simulink model "SBCAFinalSim"  (R2025b)
settings: Solver=FixedStepAuto  StartTime=0.0  StopTime=26  FixedStep=0.00005  MaxStep=0.1  RelTol=1e-3  AbsTol=1e-3  EnableMultiTasking=on
values from neighbouring files (symbols this model uses):
  K1 = lqr(A, B, Q, R_mat)    [Sim_Setup_Run_First.m]
  K2 = lqr(A, B, Q, R_mat)    [Sim_Setup_Run_First.m]
undefined symbols (not defined in the file or in its folder): X, Y, Z
libraries: sm_lib x18, nesl_utility x17
CloseFcn:
  | try,close(h1_sm_contact_ball),end
  | clear h1_sm_contact_ball
  | try,close(h2_sm_contact_ball),end
  | clear h2_sm_contact_ball
  | try,close(h3_sm_contact_ball),end
  | clear h3_sm_contact_ball
  | try,close(h4_sm_contact_ball),end
  | clear h4_sm_contact_ball
  | 
  | 
  | clear simlog_sm_contact_ball
  | clear logsout_sm_contact_ball
Description:
  | Bouncing Ball With Zero Crossings
  | 
  | Copyright 2019-2024 The MathWorks, Inc.
settings Model: Creator=smiller  LastModifiedBy=griffintrace
settings SolverCC: AutoScaleAbsTol=off  AlgebraicLoopSolver=TrustRegion  AutoInsertRateTranBlk=on
settings DataIOCC: LimitDataPoints=on  MaxDataPoints=10000  ReturnWorkspaceOutputs=off  SignalLoggingName=logsout_sm_contact_ball
settings OptimizationCC: ReuseModelBlockBuffer=off  LifeSpan=inf
settings DebuggingCC: UnconnectedInputMsg=warning  UnconnectedOutputMsg=warning  UnconnectedLineMsg=warning  AllowSymbolicDim=off  SFUnexpectedBacktrackingDiag=warning  SFNoUnconditionalDefaultTransitionDiag=warning  SFExecutionAtInitializationDiag=none  ArithmeticOperatorsInVariantConditions=warning
settings ModelReferenceCC: EnableRefExpFcnMdlSchedulingChecks=on
settings SFSimCC: SimUseLocalCustomCode=off  CustomCodeUndefinedFunction=UseInterfaceOnly
settings RTWCC: RTWUseLocalCustomCode=off  GPUComputeCapability=3.5  DLArmComputeVersion=19.05
settings CodeAppCC: StateflowObjectComments=on
settings GRTTargetCC: TargetLangStandard=C89/C90 (ANSI)
settings ConfigComp: CovMetricSettings=dw  CovSaveCumulativeToWorkspaceVar=on  CovSaveSingleToWorkspaceVar=on  CovExternalEMLEnable=off  CovSFcnEnable=off
settings SimscapeCC: SimscapeLogType=all  SimscapeLogSimulationStatistics=on  SimscapeLogName=simlog_sm_contact_ball  SimscapeLogDataHistory=10000.0
settings ExplorerConfigSet: InternalSimMechanicsExplorerSettings="<ExplorerConfiguration><canonicalview>default</canonicalview><AnimationSetting><BasePlaybackSpeed>1.0</BasePlaybackSpeed><PlaybackSpeedFactor>0.25</PlaybackSpeedFactor></AnimationSetting><TilePanel><TileInfo><Tiles Columns=\"1\" Count=\"2\" Rows=\"2\"><Column Weight=\"1\"/><Row Weight=\"0.5873\"/><Row Weight=\"0.4127\"/><Tile Height=\"1\" Width=\"1\" X=\"0\" Y=\"0\"/><Tile Height=\"1\" Width=\"1\" X=\"0\" Y=\"1\"/></Tiles></TileInfo><SceneInfo><SceneViewer><BGColor><R>1</R><G>1</G><B>1</B></BGColor><Camera><DoPerspective>off</DoPerspective><Position><X>-1.14521067233944529</X><Y>1.68242641303992024</Y><Z>0.238083627023966377</Z></Position><Center><X>-1.14521067233944529</X><Y>2.36058078639800328e-09</Y><Z>0.238083627023966377</Z></Center><Up><X>0</X><Y>0</Y><Z>1</Z></Up><ViewLimDist>1</ViewLimDist><YLim>0.433965796928594605</YLim><XLim>1.43706706523895278</XLim></Camera></SceneViewer><SceneViewer><BGColor><R>1</R><G>1</G><B>1</B></BGColor><Camera><DoPerspective>off</DoPerspective><Position><X>-1.14500851324288244</X><Y>0.00149877087782307591</Y><Z>1.68335583195827976</Z></Position><Center><X>-1.14500851324288244</X><Y>0.00149877087782307591</Y><Z>0.238083615161404305</Z></Center><Up><X>-0.00177367613036490167</X><Y>-0.9999984270352551</Y><Z>0</Z></Up><ViewLimDist>1</ViewLimDist><YLim>0.302405583873243622</YLim><XLim>1.43731595158576964</XLim></Camera></SceneViewer></SceneInfo></TilePanel><MechEditorPanel><Cameras/><GfxPanelCameraMap/><VideoCreator><PlaybackSpeedRatio>0.25</PlaybackSpeedRatio><FrameRate>30</FrameRate><VideoFormat>MPEG-4</VideoFormat><FrameSize>auto</FrameSize></VideoCreator></MechEditorPanel></ExplorerConfiguration>"

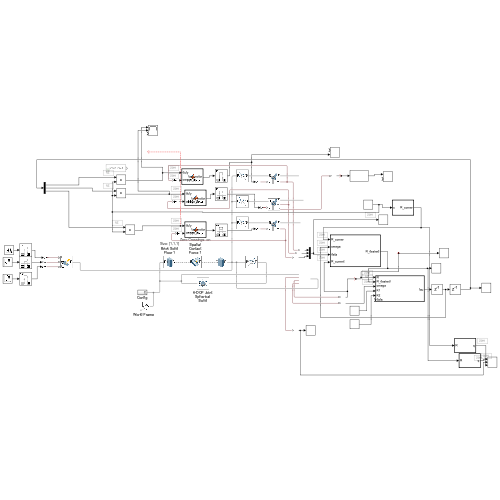
[thumbnail: Simulink's stored preview of the top-level diagram]
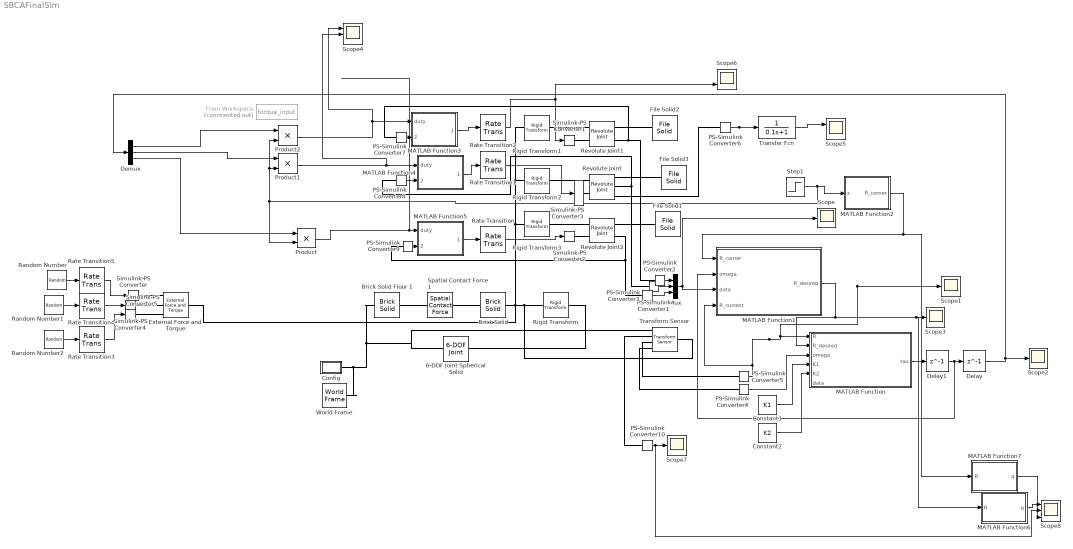
== system SBCAFinalSim ==
  6-DOF Joint Spherical Solid : sm_lib/Joints/6-DOF Joint  JointMode=Normal  CompositeWrenchDir=FollowerOnBase  CompositeWrenchFrame=BaseFrame  SenseConstraintForce=off  SenseConstraintTorque=off  SenseTotalForce=off  SenseTotalTorque=off  PxPositionTargetSpecify=off  PxPositionTargetPriority=High  PxPositionTargetValue=0  PxPositionTargetValueUnits=m  PxVelocityTargetSpecify=off  PxVelocityTargetPriority=High  PxVelocityTargetValue=0  PxVelocityTargetValueUnits=m/s  PxEquilibriumPosition=0  PxEquilibriumPositionUnits=m  PxSpringStiffness=0  PxSpringStiffnessUnits=N/m  PxDampingCoefficient=0  PxDampingCoefficientUnits=N/(m/s)  PxLowerLimitSpecify=off  PxLowerLimitBound=-1  PxLowerLimitBoundUnits=m  PxLowerLimitStiffness=1e6  PxLowerLimitStiffnessUnits=N/m  PxLowerLimitDamping=1e3  PxLowerLimitDampingUnits=N/(m/s)  PxLowerLimitTransitionRegionWidth=1e-4  PxLowerLimitTransitionRegionWidthUnits=m  PxUpperLimitSpecify=off  PxUpperLimitBound=1  PxUpperLimitBoundUnits=m  PxUpperLimitStiffness=1e6  PxUpperLimitStiffnessUnits=N/m  PxUpperLimitDamping=1e3  PxUpperLimitDampingUnits=N/(m/s)  PxUpperLimitTransitionRegionWidth=1e-4  PxUpperLimitTransitionRegionWidthUnits=m  PxTorqueActuationMode=NoTorque  PxMotionActuationMode=ComputedMotion  PxSensePosition=off  PxSenseVelocity=off  PxSenseAcceleration=off  PxSenseTorqueForce=off  PxSenseLowerLimitTorqueForce=off  PxSenseUpperLimitTorqueForce=off  PyPositionTargetSpecify=off  PyPositionTargetPriority=High  PyPositionTargetValue=0  PyPositionTargetValueUnits=m  PyVelocityTargetSpecify=off  PyVelocityTargetPriority=High  PyVelocityTargetValue=0  PyVelocityTargetValueUnits=m/s  PyEquilibriumPosition=0  PyEquilibriumPositionUnits=m  PySpringStiffness=0  PySpringStiffnessUnits=N/m  PyDampingCoefficient=0  PyDampingCoefficientUnits=N/(m/s)  PyLowerLimitSpecify=off  PyLowerLimitBound=-1  PyLowerLimitBoundUnits=m  PyLowerLimitStiffness=1e6  PyLowerLimitStiffnessUnits=N/m  PyLowerLimitDamping=1e3  PyLowerLimitDampingUnits=N/(m/s)  PyLowerLimitTransitionRegionWidth=1e-4  PyLowerLimitTransitionRegionWidthUnits=m  PyUpperLimitSpecify=off  PyUpperLimitBound=1  PyUpperLimitBoundUnits=m  PyUpperLimitStiffness=1e6  PyUpperLimitStiffnessUnits=N/m  PyUpperLimitDamping=1e3  PyUpperLimitDampingUnits=N/(m/s)  PyUpperLimitTransitionRegionWidth=1e-4  PyUpperLimitTransitionRegionWidthUnits=m  PyTorqueActuationMode=NoTorque  PyMotionActuationMode=ComputedMotion  PySensePosition=off  PySenseVelocity=off  PySenseAcceleration=off  PySenseTorqueForce=off  PySenseLowerLimitTorqueForce=off  PySenseUpperLimitTorqueForce=off  PzPositionTargetSpecify=on  PzPositionTargetPriority=High  PzPositionTargetValue=0.45  PzPositionTargetValueUnits=m  PzVelocityTargetSpecify=off  PzVelocityTargetPriority=High  PzVelocityTargetValue=0  PzVelocityTargetValueUnits=m/s  PzEquilibriumPosition=0  PzEquilibriumPositionUnits=m  PzSpringStiffness=0  PzSpringStiffnessUnits=N/m  PzDampingCoefficient=0  PzDampingCoefficientUnits=N/(m/s)  PzLowerLimitSpecify=off  PzLowerLimitBound=-1  PzLowerLimitBoundUnits=m  PzLowerLimitStiffness=1e6  PzLowerLimitStiffnessUnits=N/m  PzLowerLimitDamping=1e3  PzLowerLimitDampingUnits=N/(m/s)  PzLowerLimitTransitionRegionWidth=1e-4  PzLowerLimitTransitionRegionWidthUnits=m  PzUpperLimitSpecify=off  PzUpperLimitBound=1  PzUpperLimitBoundUnits=m  PzUpperLimitStiffness=1e6  PzUpperLimitStiffnessUnits=N/m  PzUpperLimitDamping=1e3  PzUpperLimitDampingUnits=N/(m/s)  PzUpperLimitTransitionRegionWidth=1e-4  PzUpperLimitTransitionRegionWidthUnits=m  PzTorqueActuationMode=NoTorque  PzMotionActuationMode=ComputedMotion  PzSensePosition=off  PzSenseVelocity=off  PzSenseAcceleration=off  PzSenseTorqueForce=off  PzSenseLowerLimitTorqueForce=off  PzSenseUpperLimitTorqueForce=off  SphPositionTargetSpecify=off  SphPositionTargetPriority=High  SphPositionTargetRotationMethod=None  SphPositionTargetFollAlignAxisA=+X  SphPositionTargetBaseAlignAxisA=+Y  SphPositionTargetFollAlignAxisB=+Y  SphPositionTargetBaseAlignAxisB=+Z  SphPositionTargetRotationStandardAxis=+Z  SphPositionTargetRotationAngle=0.0  SphPositionTargetRotationAngleUnits=deg  SphPositionTargetRotationArbitraryAxis=[0 0 1]  SphPositionTargetRotationSequenceAxes=FollowerAxes  SphPositionTargetRotationSequence=XYX  SphPositionTargetRotationSequenceAngles=[0 0 0]  SphPositionTargetRotationSequenceAnglesUnits=deg  SphPositionTargetRotationMatrix=[1 0 0; 0 1 0; 0 0 1]  SphPositionTargetQuaternion=[1 0 0 0]  SphVelocityTargetSpecify=off  SphVelocityTargetPriority=High  SphVelocityTargetValue=[0 0 0]  SphVelocityTargetValueUnits=deg/s  SphVelocityTargetInFollowerFrame=on  SphEqPosRotationMethod=None  SphEqPosFollAlignAxisA=+X  SphEqPosBaseAlignAxisA=+Y  SphEqPosFollAlignAxisB=+Y  SphEqPosBaseAlignAxisB=+Z  SphEqPosRotationStandardAxis=+Z  SphEqPosRotationAngle=0.0  SphEqPosRotationAngleUnits=deg  SphEqPosRotationArbitraryAxis=[0 0 1]  SphEqPosRotationSequenceAxes=FollowerAxes  SphEqPosRotationSequence=XYX  SphEqPosRotationSequenceAngles=[0 0 0]  SphEqPosRotationSequenceAnglesUnits=deg  SphEqPosRotationMatrix=[1 0 0; 0 1 0; 0 0 1]  SphEqPosQuaternion=[1 0 0 0]  SphSpringStiffness=0  SphSpringStiffnessUnits=N*m/deg  SphDampingCoefficient=0  SphDampingCoefficientUnits=N*m/(deg/s)  SphLowerLimitSpecify=off  SphLowerLimitBound=15  SphLowerLimitBoundUnits=deg  SphLowerLimitStiffness=1e4  SphLowerLimitStiffnessUnits=N*m/deg  SphLowerLimitDamping=10  SphLowerLimitDampingUnits=N*m/(deg/s)  SphLowerLimitTransitionRegionWidth=0.1  SphLowerLimitTransitionRegionWidthUnits=deg  SphUpperLimitSpecify=off  SphUpperLimitBound=45  SphUpperLimitBoundUnits=deg  SphUpperLimitStiffness=1e4  SphUpperLimitStiffnessUnits=N*m/deg  SphUpperLimitDamping=10  SphUpperLimitDampingUnits=N*m/(deg/s)  SphUpperLimitTransitionRegionWidth=0.1  SphUpperLimitTransitionRegionWidthUnits=deg  SphTorqueActuationMode=NoTorque  SphActuateTorqueX=off  SphActuateTorqueY=off  SphActuateTorqueZ=off  SphActuateTorque=off  SphActuationFrame=BaseFrame  SphSensePosition=off  SphSenseVelocityX=off  SphSenseVelocityY=off  SphSenseVelocityZ=off  SphSenseVelocity=off  SphSenseAccelerationX=off  SphSenseAccelerationY=off  SphSenseAccelerationZ=off  SphSenseAcceleration=off  SphSenseLowerLimitTorqueMag=off  SphSenseUpperLimitTorqueMag=off  SphSensingFrame=BaseFrame
  Brick Solid : sm_lib/Body Elements/Brick Solid  BrickDimensions=[0.124 0.124 0.124]  BrickDimensionsUnits=m  ExportEntireGeometry=on  InertiaType=Custom  BasedOnType=Mass  Density=1000  DensityUnits=kg/m^3  Mass=0.374  MassUnits=kg  CenterOfMass=[-20 -20 -20]  CenterOfMassUnits=mm  MomentsOfInertia=[0.0011441 0.0011441 0.0011441]  MomentsOfInertiaUnits=kg*m^2  ProductsOfInertia=[0.00018195 0.00018195 0.00018195]  ProductsOfInertiaUnits=kg*m^2  GraphicType=FromGeometry  MarkerShape=Sphere  MarkerSize=10  GraphicVisPropType=SimpleVisualProperties  GraphicDiffuseColor=[1 0 0]  GraphicOpacity=0.2  GraphicSpecularColor=[0.5 0.5 0.5 1.0]  GraphicAmbientColor=[0.15 0.15 0.15 1.0]  GraphicEmissiveColor=[0.0 0.0 0.0 1.0]  GraphicShininess=75  DoExposeReferenceFrame=on  SerializedFrames=<Frames/>
  Brick Solid Floor 1 : sm_lib/Body Elements/Brick Solid  BrickDimensions=[1,1,1]  BrickDimensionsUnits=m  ExportEntireGeometry=on  InertiaType=CalculateFromGeometry  BasedOnType=Density  Density=1000  DensityUnits=kg/m^3  Mass=1  MassUnits=kg  CenterOfMass=[0 0 0]  CenterOfMassUnits=m  MomentsOfInertia=[1 1 1]  MomentsOfInertiaUnits=kg*m^2  ProductsOfInertia=[0 0 0]  ProductsOfInertiaUnits=kg*m^2  GraphicType=FromGeometry  MarkerShape=Sphere  MarkerSize=10  GraphicVisPropType=SimpleVisualProperties  GraphicDiffuseColor=[0.7882 1 0.9725]  GraphicOpacity=1.0  GraphicSpecularColor=[0.5 0.5 0.5 1.0]  GraphicAmbientColor=[0.15 0.15 0.15 1.0]  GraphicEmissiveColor=[0.0 0.0 0.0 1.0]  GraphicShininess=75  DoExposeReferenceFrame=off  SerializedFrames=<Frames><Frame><Id>Frame1</Id><Value><Name>F1</Name><Origin><Source>ReferenceFrame</Source><FeatureName></FeatureName></Origin><PrimaryAxis><DefinedDirection>+Z</DefinedDirection><Source>ReferenceFrame</Source><SourceDirection>+Z</SourceDirection><FeatureName></FeatureName></PrimaryAxis><SecondaryAxis><DefinedDirection>+X</DefinedDirection><Source>ReferenceFrame</Source><SourceDirection>+X</SourceDirection><FeatureName></FeatureName></SecondaryAxis></Value></Frame></Frames>
      settings: AttributesFormatString=Size: %<BrickDimensions>
  Config : Subsystem
  Constant1 : Constant  Value=K1
  Constant2 : Constant  Value=K2
  Delay : Delay  DelayLength=1
  Delay1 : Delay  DelayLength=1
  Demux : Demux  Outputs=3
  External Force and Torque : sm_lib/Forces and Torques/External Force and Torque  EnableForceX=off  EnableForceY=off  EnableForceZ=off  EnableForce=off  ForceResolutionFrame=AttachedFrame  EnableTorqueX=on  EnableTorqueY=on  EnableTorqueZ=on  EnableTorque=off  TorqueResolutionFrame=AttachedFrame
  File Solid1 : sm_lib/Body Elements/File Solid  ExtGeomFileName=/Users/griffintrace/Downloads/Part Studio 1 - Wheel 1.step  UnitType=FromFile  ExtGeomFileUnits=m  StepReaderType=HEX  ExportConvexHullGeometry=off  InertiaType=Custom  BasedOnType=DensityFromFile  Density=1000  DensityUnits=kg/m^3  Mass=0.051  MassUnits=kg  CenterOfMass=[0 0 0]  CenterOfMassUnits=m  MomentsOfInertia=[0.00004749 0.00004749 0.00009362]  MomentsOfInertiaUnits=kg*m^2  ProductsOfInertia=[0 0 0]  ProductsOfInertiaUnits=kg*m^2  GraphicType=FromGeometry  MarkerShape=Sphere  MarkerSize=10  GraphicVisPropType=SimpleVisualProperties  GraphicDiffuseColor=[0.5 0.5 0.5]  GraphicOpacity=1  GraphicSpecularColor=[0.5 0.5 0.5 1.0]  GraphicAmbientColor=[0.15 0.15 0.15 1.0]  GraphicEmissiveColor=[0.0 0.0 0.0 1.0]  GraphicShininess=75  DoExposeReferenceFrame=on  SerializedFrames=<Frames/>
  File Solid2 : sm_lib/Body Elements/File Solid  ExtGeomFileName=/Users/griffintrace/Downloads/Part Studio 1 - Wheel 1.step  UnitType=FromFile  ExtGeomFileUnits=m  StepReaderType=HEX  ExportConvexHullGeometry=off  InertiaType=Custom  BasedOnType=DensityFromFile  Density=1000  DensityUnits=kg/m^3  Mass=0.051  MassUnits=kg  CenterOfMass=[0 0 0]  CenterOfMassUnits=m  MomentsOfInertia=[0.00004749 0.00004749 0.00009362]  MomentsOfInertiaUnits=kg*m^2  ProductsOfInertia=[0 0 0]  ProductsOfInertiaUnits=kg*m^2  GraphicType=FromGeometry  MarkerShape=Sphere  MarkerSize=10  GraphicVisPropType=SimpleVisualProperties  GraphicDiffuseColor=[0.5 0.5 0.5]  GraphicOpacity=1  GraphicSpecularColor=[0.5 0.5 0.5 1.0]  GraphicAmbientColor=[0.15 0.15 0.15 1.0]  GraphicEmissiveColor=[0.0 0.0 0.0 1.0]  GraphicShininess=75  DoExposeReferenceFrame=on  SerializedFrames=<Frames/>
  File Solid3 : sm_lib/Body Elements/File Solid  ExtGeomFileName=/Users/griffintrace/Downloads/Part Studio 1 - Wheel 1.step  UnitType=FromFile  ExtGeomFileUnits=m  StepReaderType=HEX  ExportConvexHullGeometry=off  InertiaType=Custom  BasedOnType=DensityFromFile  Density=1000  DensityUnits=kg/m^3  Mass=0.051  MassUnits=kg  CenterOfMass=[0 0 0]  CenterOfMassUnits=m  MomentsOfInertia=[0.00004749 0.00004749 0.00009362]  MomentsOfInertiaUnits=kg*m^2  ProductsOfInertia=[0 0 0]  ProductsOfInertiaUnits=kg*m^2  GraphicType=FromGeometry  MarkerShape=Sphere  MarkerSize=10  GraphicVisPropType=SimpleVisualProperties  GraphicDiffuseColor=[0.5 0.5 0.5]  GraphicOpacity=1  GraphicSpecularColor=[0.5 0.5 0.5 1.0]  GraphicAmbientColor=[0.15 0.15 0.15 1.0]  GraphicEmissiveColor=[0.0 0.0 0.0 1.0]  GraphicShininess=75  DoExposeReferenceFrame=on  SerializedFrames=<Frames/>
  From Workspace : FromWorkspace  Commented=on  VariableName=torque_input  SampleTime=-1
  MATLAB Function : MATLAB Function  TreatAsAtomicUnit=on  SystemSampleTime=0.0005
  MATLAB Function1 : MATLAB Function  TreatAsAtomicUnit=on  SystemSampleTime=0.001
  MATLAB Function2 : MATLAB Function  TreatAsAtomicUnit=on
  MATLAB Function3 : MATLAB Function  TreatAsAtomicUnit=on  SystemSampleTime=0.0001
  MATLAB Function4 : MATLAB Function  TreatAsAtomicUnit=on  SystemSampleTime=0.0001
  MATLAB Function5 : MATLAB Function  TreatAsAtomicUnit=on  SystemSampleTime=0.0001
  MATLAB Function6 : MATLAB Function  TreatAsAtomicUnit=on
  MATLAB Function7 : MATLAB Function  TreatAsAtomicUnit=on
  Mux : Mux  Inputs=3
  PS-Simulink Converter{1..10} (10 alike) : nesl_utility/PS-Simulink Converter  PhysicalDomain=network_engine_domain  SubClassName=ps_output  LeftPortType=input  RightPortType=output  PseudoPeriodic=off  Frequencies=[]  VectorFormat=inherit  Unit=inherit  AffineConversion=off
  Product : Product
  Product1 : Product
  Product2 : Product
  Random Number : RandomNumber  Variance=0.01  SampleTime=0.001
  Random Number1 : RandomNumber  Variance=0.01  Seed=10000  SampleTime=0.001
  Random Number2 : RandomNumber  Variance=0.01  Seed=10  SampleTime=0.001
  Rate Transition{,1..5} (6 alike) : RateTransition
  Revolute Joint : sm_lib/Joints/Revolute Joint  JointMode=Normal  CompositeWrenchDir=FollowerOnBase  CompositeWrenchFrame=BaseFrame  SenseConstraintForce=off  SenseConstraintTorque=off  SenseTotalForce=off  SenseTotalTorque=off  PositionTargetSpecify=off  PositionTargetPriority=High  PositionTargetValue=0  PositionTargetValueUnits=deg  VelocityTargetSpecify=off  VelocityTargetPriority=High  VelocityTargetValue=0  VelocityTargetValueUnits=deg/s  EquilibriumPosition=0  EquilibriumPositionUnits=deg  SpringStiffness=0  SpringStiffnessUnits=N*m/deg  DampingCoefficient=0  DampingCoefficientUnits=N*m/(deg/s)  LowerLimitSpecify=off  LowerLimitBound=-90  LowerLimitBoundUnits=deg  LowerLimitStiffness=1e4  LowerLimitStiffnessUnits=N*m/deg  LowerLimitDamping=10  LowerLimitDampingUnits=N*m/(deg/s)  LowerLimitTransitionRegionWidth=0.1  LowerLimitTransitionRegionWidthUnits=deg  UpperLimitSpecify=off  UpperLimitBound=90  UpperLimitBoundUnits=deg  UpperLimitStiffness=1e4  UpperLimitStiffnessUnits=N*m/deg  UpperLimitDamping=10  UpperLimitDampingUnits=N*m/(deg/s)  UpperLimitTransitionRegionWidth=0.1  UpperLimitTransitionRegionWidthUnits=deg  TorqueActuationMode=InputTorque  MotionActuationMode=ComputedMotion  SensePosition=off  SenseVelocity=on  SenseAcceleration=off  SenseTorqueForce=on  SenseLowerLimitTorqueForce=off  SenseUpperLimitTorqueForce=off
  Revolute Joint1 : sm_lib/Joints/Revolute Joint  JointMode=Normal  CompositeWrenchDir=FollowerOnBase  CompositeWrenchFrame=BaseFrame  SenseConstraintForce=off  SenseConstraintTorque=off  SenseTotalForce=off  SenseTotalTorque=off  PositionTargetSpecify=off  PositionTargetPriority=High  PositionTargetValue=0  PositionTargetValueUnits=deg  VelocityTargetSpecify=off  VelocityTargetPriority=High  VelocityTargetValue=0  VelocityTargetValueUnits=deg/s  EquilibriumPosition=0  EquilibriumPositionUnits=deg  SpringStiffness=0  SpringStiffnessUnits=N*m/deg  DampingCoefficient=0  DampingCoefficientUnits=N*m/(deg/s)  LowerLimitSpecify=off  LowerLimitBound=-90  LowerLimitBoundUnits=deg  LowerLimitStiffness=1e4  LowerLimitStiffnessUnits=N*m/deg  LowerLimitDamping=10  LowerLimitDampingUnits=N*m/(deg/s)  LowerLimitTransitionRegionWidth=0.1  LowerLimitTransitionRegionWidthUnits=deg  UpperLimitSpecify=off  UpperLimitBound=90  UpperLimitBoundUnits=deg  UpperLimitStiffness=1e4  UpperLimitStiffnessUnits=N*m/deg  UpperLimitDamping=10  UpperLimitDampingUnits=N*m/(deg/s)  UpperLimitTransitionRegionWidth=0.1  UpperLimitTransitionRegionWidthUnits=deg  TorqueActuationMode=InputTorque  MotionActuationMode=ComputedMotion  SensePosition=off  SenseVelocity=on  SenseAcceleration=off  SenseTorqueForce=off  SenseLowerLimitTorqueForce=off  SenseUpperLimitTorqueForce=off
  Revolute Joint2 : sm_lib/Joints/Revolute Joint  JointMode=Normal  CompositeWrenchDir=FollowerOnBase  CompositeWrenchFrame=BaseFrame  SenseConstraintForce=off  SenseConstraintTorque=off  SenseTotalForce=off  SenseTotalTorque=off  PositionTargetSpecify=off  PositionTargetPriority=High  PositionTargetValue=0  PositionTargetValueUnits=deg  VelocityTargetSpecify=off  VelocityTargetPriority=High  VelocityTargetValue=0  VelocityTargetValueUnits=deg/s  EquilibriumPosition=0  EquilibriumPositionUnits=deg  SpringStiffness=0  SpringStiffnessUnits=N*m/deg  DampingCoefficient=0  DampingCoefficientUnits=N*m/(deg/s)  LowerLimitSpecify=off  LowerLimitBound=-90  LowerLimitBoundUnits=deg  LowerLimitStiffness=1e4  LowerLimitStiffnessUnits=N*m/deg  LowerLimitDamping=10  LowerLimitDampingUnits=N*m/(deg/s)  LowerLimitTransitionRegionWidth=0.1  LowerLimitTransitionRegionWidthUnits=deg  UpperLimitSpecify=off  UpperLimitBound=90  UpperLimitBoundUnits=deg  UpperLimitStiffness=1e4  UpperLimitStiffnessUnits=N*m/deg  UpperLimitDamping=10  UpperLimitDampingUnits=N*m/(deg/s)  UpperLimitTransitionRegionWidth=0.1  UpperLimitTransitionRegionWidthUnits=deg  TorqueActuationMode=InputTorque  MotionActuationMode=ComputedMotion  SensePosition=off  SenseVelocity=on  SenseAcceleration=off  SenseTorqueForce=off  SenseLowerLimitTorqueForce=off  SenseUpperLimitTorqueForce=off
  Rigid Transform : sm_lib/Frames and Transforms/Rigid Transform  RotationMethod=StandardAxis  FollAlignAxisA=+X  BaseAlignAxisA=+Y  FollAlignAxisB=+Y  BaseAlignAxisB=+Z  RotationStandardAxis=+Y  RotationAngle=0  RotationAngleUnits=deg  RotationArbitraryAxis=[0 0 1]  RotationSequenceAxes=FollowerAxes  RotationSequence=XYX  RotationSequenceAngles=[0 0 0]  RotationSequenceAnglesUnits=deg  RotationMatrix=[1 0 0;0 1 0;0 0 1]  Quaternion=[1 0 0 0]  TranslationMethod=StandardAxis  TranslationCartesianOffset=[0 0 0]  TranslationCartesianOffsetUnits=m  TranslationStandardAxis=+Z  TranslationStandardOffset=-0.112  TranslationStandardOffsetUnits=m  TranslationROffset=0  TranslationROffsetUnits=m  TranslationThetaOffset=0  TranslationThetaOffsetUnits=deg  TranslationZOffset=0  TranslationZOffsetUnits=m
  Rigid Transform1 : sm_lib/Frames and Transforms/Rigid Transform  RotationMethod=StandardAxis  FollAlignAxisA=+X  BaseAlignAxisA=+Y  FollAlignAxisB=+Y  BaseAlignAxisB=+Z  RotationStandardAxis=-Y  RotationAngle=90  RotationAngleUnits=deg  RotationArbitraryAxis=[0 0 1]  RotationSequenceAxes=FollowerAxes  RotationSequence=XYX  RotationSequenceAngles=[0 0 0]  RotationSequenceAnglesUnits=deg  RotationMatrix=[1 0 0;0 1 0;0 0 1]  Quaternion=[1 0 0 0]  TranslationMethod=Cartesian  TranslationCartesianOffset=[0 0 0.055]  TranslationCartesianOffsetUnits=m  TranslationStandardAxis=+Z  TranslationStandardOffset=0  TranslationStandardOffsetUnits=m  TranslationROffset=0  TranslationROffsetUnits=m  TranslationThetaOffset=0  TranslationThetaOffsetUnits=deg  TranslationZOffset=0  TranslationZOffsetUnits=m
  Rigid Transform2 : sm_lib/Frames and Transforms/Rigid Transform  RotationMethod=StandardAxis  FollAlignAxisA=+X  BaseAlignAxisA=+Y  FollAlignAxisB=+Y  BaseAlignAxisB=+Z  RotationStandardAxis=+X  RotationAngle=90  RotationAngleUnits=deg  RotationArbitraryAxis=[0 0 1]  RotationSequenceAxes=FollowerAxes  RotationSequence=XYX  RotationSequenceAngles=[0 0 0]  RotationSequenceAnglesUnits=deg  RotationMatrix=[1 0 0;0 1 0;0 0 1]  Quaternion=[1 0 0 0]  TranslationMethod=Cartesian  TranslationCartesianOffset=[0 0 0.055]  TranslationCartesianOffsetUnits=m  TranslationStandardAxis=+Z  TranslationStandardOffset=0  TranslationStandardOffsetUnits=m  TranslationROffset=0  TranslationROffsetUnits=m  TranslationThetaOffset=0  TranslationThetaOffsetUnits=deg  TranslationZOffset=0  TranslationZOffsetUnits=m
  Rigid Transform3 : sm_lib/Frames and Transforms/Rigid Transform  RotationMethod=StandardAxis  FollAlignAxisA=+X  BaseAlignAxisA=+Y  FollAlignAxisB=+Y  BaseAlignAxisB=+Z  RotationStandardAxis=-Z  RotationAngle=90  RotationAngleUnits=deg  RotationArbitraryAxis=[0 0 1]  RotationSequenceAxes=FollowerAxes  RotationSequence=XYX  RotationSequenceAngles=[0 0 0]  RotationSequenceAnglesUnits=deg  RotationMatrix=[1 0 0;0 1 0;0 0 1]  Quaternion=[1 0 0 0]  TranslationMethod=Cartesian  TranslationCartesianOffset=[0 0 0.055]  TranslationCartesianOffsetUnits=m  TranslationStandardAxis=+Z  TranslationStandardOffset=0  TranslationStandardOffsetUnits=m  TranslationROffset=0  TranslationROffsetUnits=m  TranslationThetaOffset=0  TranslationThetaOffsetUnits=deg  TranslationZOffset=0  TranslationZOffsetUnits=m
  Scope{,1..3,7} (5 alike) : Scope
      Scope settings: SampleTime=0.01  ActiveDisplayYMinimum=-606.88398  ActiveDisplayYMaximum=752.93887  DataLoggingVariableName=RPM
      Scope1 settings: ActiveDisplayYMinimum=-0.95959  ActiveDisplayYMaximum=1.21773  DataLoggingVariableName=ScopeData2
      Scope2 settings: ActiveDisplayYMinimum=-1.25  ActiveDisplayYMaximum=1.25
      Scope3 settings: ActiveDisplayYMinimum=-1.78359  ActiveDisplayYMaximum=1.88444  DataLoggingVariableName=ScopeData3
      Scope7 settings: ActiveDisplayYMinimum=-1.25  ActiveDisplayYMaximum=1.25
  Scope4 : Scope  NumInputPorts=3
      settings: ActiveDisplayYMinimum=-0.125  ActiveDisplayYMaximum=1.125
  Scope5 : Scope  NumInputPorts=2
      settings: ActiveDisplayYMinimum=-0.79406  ActiveDisplayYMaximum=0.62384  DataLoggingVariableName=ScopeData2
  Scope6 : Scope  NumInputPorts=2
      settings: ActiveDisplayYMinimum=-0.3668  ActiveDisplayYMaximum=0.36762  DataLoggingVariableName=ScopeData3
  Scope8 : Scope  NumInputPorts=3
      settings: SampleTime=0.01  ActiveDisplayYMinimum=-0.61104  ActiveDisplayYMaximum=1.179  DataLoggingVariableName=PosSim
  Simulink-PS Converter : nesl_utility/Simulink-PS Converter  PhysicalDomain=network_engine_domain  SubClassName=ps_input  LeftPortType=input  RightPortType=output  PseudoPeriodic=off  Frequencies=[]  NoiseDistribution=none  NoiseParameters=[]  Unit=1  AffineConversion=off  FilteringAndDerivatives=filter  SimscapeFilterOrder=1  InputFilterTimeConstant=0.1  UdotUserProvided=0
  Simulink-PS Converter1 : nesl_utility/Simulink-PS Converter  PhysicalDomain=network_engine_domain  SubClassName=ps_input  LeftPortType=input  RightPortType=output  PseudoPeriodic=off  Frequencies=[]  NoiseDistribution=none  NoiseParameters=[]  Unit=1  AffineConversion=off  FilteringAndDerivatives=provide  SimscapeFilterOrder=2  InputFilterTimeConstant=0.0001  UdotUserProvided=0
  Simulink-PS Converter2 : nesl_utility/Simulink-PS Converter  PhysicalDomain=network_engine_domain  SubClassName=ps_input  LeftPortType=input  RightPortType=output  PseudoPeriodic=off  Frequencies=[]  NoiseDistribution=none  NoiseParameters=[]  Unit=1  AffineConversion=off  FilteringAndDerivatives=provide  SimscapeFilterOrder=2  InputFilterTimeConstant=0.0001  UdotUserProvided=0
  Simulink-PS Converter3 : nesl_utility/Simulink-PS Converter  PhysicalDomain=network_engine_domain  SubClassName=ps_input  LeftPortType=input  RightPortType=output  PseudoPeriodic=off  Frequencies=[]  NoiseDistribution=none  NoiseParameters=[]  Unit=1  AffineConversion=off  FilteringAndDerivatives=provide  SimscapeFilterOrder=2  InputFilterTimeConstant=0.0001  UdotUserProvided=0
  Simulink-PS Converter4 : nesl_utility/Simulink-PS Converter  PhysicalDomain=network_engine_domain  SubClassName=ps_input  LeftPortType=input  RightPortType=output  PseudoPeriodic=off  Frequencies=[]  NoiseDistribution=none  NoiseParameters=[]  Unit=1  AffineConversion=off  FilteringAndDerivatives=filter  SimscapeFilterOrder=1  InputFilterTimeConstant=0.1  UdotUserProvided=0
  Simulink-PS Converter5 : nesl_utility/Simulink-PS Converter  PhysicalDomain=network_engine_domain  SubClassName=ps_input  LeftPortType=input  RightPortType=output  PseudoPeriodic=off  Frequencies=[]  NoiseDistribution=none  NoiseParameters=[]  Unit=1  AffineConversion=off  FilteringAndDerivatives=filter  SimscapeFilterOrder=1  InputFilterTimeConstant=0.1  UdotUserProvided=0
  Spatial Contact Force 1 : sm_lib/Forces and Torques/Spatial Contact Force  SenseSeparationDistance=off  NormalForceType=SmoothSpringDamper  NormalStiffness=1e7  NormalStiffnessUnits=N/m  NormalDamping=10e3  NormalDampingUnits=N/(m/s)  NormalTransitionRegionWidth=5e-2  NormalTransitionRegionWidthUnits=m  FrictionType=SmoothStickSlip  CoefficientOfStaticFriction=1  CoefficientOfDynamicFriction=1  FrictionalCriticalVelocity=1e-3  FrictionalCriticalVelocityUnits=m/s  SenseContactSignal=off  SensePenetrationDepth=off  SenseNormalVelocity=off  SenseTangentialVelocity=off  SensingForceTorqueDirection=BaseOnFollower  SensingForceTorqueResolutionFrame=ContactFrame  SenseNormalForce=off  SenseNormalForceMagnitude=off  SenseNormalTorque=off  SenseFrictionalForce=off  SenseFrictionalForceMagnitude=off  SenseFrictionalTorque=off  SenseTotalForce=off  SenseTotalTorque=off  SenseContactBaseRotation=off  SenseContactBaseTranslation=off  SenseContactFollowerRotation=off  SenseContactFollowerTranslation=off  ZeroCrossDetectContactStartAndEnd=on
      settings: AttributesFormatString=Zero Crossings: %<ZeroCrossDetectContactStartAndEnd>
  Step1 : Step  SampleTime=0
  Transfer Fcn : TransferFcn  Denominator=[0.1 1]
  Transform Sensor : sm_lib/Frames and Transforms/Transform Sensor  MeasurementFrame=World  RotationSequence=XYZ  SenseAngle=off  SenseAxis=off  SenseQ=on  SenseR=on  SenseRotationSequence=off  SenseOmegaX=off  SenseOmegaY=off  SenseOmegaZ=off  SenseOmega=on  SenseQDot=off  SenseRDot=off  SenseRotationSequenceDot=off  SenseAlphaX=off  SenseAlphaY=off  SenseAlphaZ=off  SenseAlpha=off  SenseQDDot=off  SenseRDDot=off  SenseX=off  SenseY=off  SenseZ=off  SenseXYZ=off  SenseRad=off  SenseAzim=off  SenseDist=off  SenseInc=off  SenseXDot=off  SenseYDot=off  SenseZDot=off  SenseXYZDot=off  SenseRadDot=off  SenseAzimDot=off  SenseDistDot=off  SenseIncDot=off  SenseXDDot=off  SenseYDDot=off  SenseZDDot=off  SenseXYZDDot=off  SenseRadDDot=off  SenseAzimDDot=off  SenseDistDDot=off  SenseIncDDot=off
  World Frame : sm_lib/Frames and Transforms/World Frame
  wires:
  PS-Simulink Converter1/1 -> Mux/2
  PS-Simulink Converter5/1 -> Scope1/1, MATLAB Function/1(R), MATLAB Function1/4(R_current)
  Mux/1 -> Scope/1, MATLAB Function1/3(data)
  PS-Simulink Converter2/1 -> Mux/1
  PS-Simulink Converter3/1 -> Mux/3
  PS-Simulink Converter4/1 -> MATLAB Function/3(omega)
  MATLAB Function1/1(R_desired) -> MATLAB Function/2(R_desired), MATLAB Function6/1(R), Scope3/1
  MATLAB Function2/1(R_corner) -> MATLAB Function7/1(R), MATLAB Function1/1(R_corner)
  Step1/1 -> Product/2, Product1/2, Product2/2, MATLAB Function2/1(x)
  MATLAB Function3/1(tau_motor) -> Rate Transition2/1
  Rate Transition/1 -> Simulink-PS Converter2/1
  Rate Transition2/1 -> Simulink-PS Converter1/1, Scope6/2
  MATLAB Function4/1(tau_motor) -> Rate Transition1/1
  MATLAB Function5/1(tau_motor) -> Rate Transition/1
  PS-Simulink Converter6/1 -> Transfer Fcn/1
  Rate Transition1/1 -> Simulink-PS Converter3/1
  Transfer Fcn/1 -> Scope5/1
  PS-Simulink Converter7/1 -> MATLAB Function3/2(omega_w)
  PS-Simulink Converter8/1 -> MATLAB Function4/2(omega_w)
  PS-Simulink Converter9/1 -> MATLAB Function5/2(omega_w)
  PS-Simulink Converter10/1 -> Scope8/2, Scope7/1
  Delay/1 -> Demux/1, Scope2/1
  Demux/3 -> Product/1
  Demux/2 -> Product1/1
  Demux/1 -> Product2/1
  Product2/1 -> Scope4/1, MATLAB Function3/1(duty)
  Product1/1 -> MATLAB Function4/1(duty), Scope4/2
  Product/1 -> MATLAB Function5/1(duty)
  Constant1/1 -> MATLAB Function/4(K1)
  Constant2/1 -> MATLAB Function/5(K2)
  Delay1/1 -> MATLAB Function1/2(omega), Delay/1
  MATLAB Function/1(tau) -> Delay1/1
  Random Number/1 -> Rate Transition5/1
  Random Number1/1 -> Rate Transition4/1
  Random Number2/1 -> Rate Transition3/1
  Rate Transition3/1 -> Simulink-PS Converter5/1
  Rate Transition4/1 -> Simulink-PS Converter4/1
  Rate Transition5/1 -> Simulink-PS Converter/1
  MATLAB Function6/1(q) -> Scope8/1
  MATLAB Function7/1(q) -> Scope8/3
  connections:
  World Frame/RConn1 -- 6-DOF Joint Spherical Solid/LConn1 -- Transform Sensor/RConn1 -- Brick Solid Floor 1/LConn1 -- Config/RConn1
  Spatial Contact Force 1/RConn1 -- Brick Solid/LConn1
  Rigid Transform/LConn1 -- External Force and Torque/RConn1 -- Brick Solid/RConn1 -- Rigid Transform3/RConn1 -- Rigid Transform1/RConn1 -- Rigid Transform2/RConn1 -- Transform Sensor/LConn1
  Rigid Transform/RConn1 -- 6-DOF Joint Spherical Solid/RConn1
  Brick Solid Floor 1/RConn1 -- Spatial Contact Force 1/LConn1
  File Solid3/RConn1 -- Revolute Joint/RConn1
  Simulink-PS Converter3/RConn1 -- Revolute Joint/LConn2
  Revolute Joint/RConn2 -- PS-Simulink Converter8/LConn1 -- PS-Simulink Converter1/LConn1
  Rigid Transform2/LConn1 -- Revolute Joint/LConn1
  Transform Sensor/RConn3 -- PS-Simulink Converter5/LConn1
  Transform Sensor/RConn4 -- PS-Simulink Converter4/LConn1
  File Solid2/RConn1 -- Revolute Joint1/RConn1
  Rigid Transform1/LConn1 -- Revolute Joint1/LConn1
  PS-Simulink Converter2/LConn1 -- PS-Simulink Converter7/LConn1 -- Revolute Joint1/RConn2
  Simulink-PS Converter1/RConn1 -- Revolute Joint1/LConn2
  File Solid1/RConn1 -- Revolute Joint2/RConn1
  Rigid Transform3/LConn1 -- Revolute Joint2/LConn1
  Revolute Joint2/RConn2 -- PS-Simulink Converter9/LConn1 -- PS-Simulink Converter3/LConn1
  Simulink-PS Converter2/RConn1 -- Revolute Joint2/LConn2
  Revolute Joint/RConn3 -- PS-Simulink Converter6/LConn1
  Transform Sensor/RConn2 -- PS-Simulink Converter10/LConn1
  Simulink-PS Converter/RConn1 -- External Force and Torque/LConn1
  Simulink-PS Converter5/RConn1 -- External Force and Torque/LConn3
  Simulink-PS Converter4/RConn1 -- External Force and Torque/LConn2

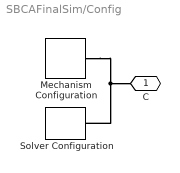
== system SBCAFinalSim/Config ==
  Mechanism Configuration : sm_lib/Utilities/Mechanism Configuration  UniformGravity=Constant  GravityVector=[0 0 -9.80665]  GravityVectorUnits=m/s^2  LinearizationDelta=0.001  JointModeTransitionNonlinearIterations=2
  Solver Configuration : nesl_utility/Solver Configuration  PhysicalDomain=network_engine_domain  SubClassName=solver  LeftPortType=input  RightPortType=generic  Tones=[]  Harmonics=[]  SimulateNoise=off  Profile=off  UseLocalSampling=off  EnableSwitchedLinearOptims=on  FrequencyDomain=off  UseCCode=off  RelTol=0.001  AbsTol=1e-06  MinStep=1e-09  ToWorkspace=off  RevertToSquareIcSolve=off  NumHomotopyIterations=100  PhasorMode=off  PhasorModeNumHarmonics=1  ConsistencySolver=NEWTON_FTOL  IndexReductionMethod=DerivativeReplacement  DoDC=off  ResidualTolerance=1e-09  ConsistencyTolSource=GLOBAL  ConsistencyAbsTol=0.001  ConsistencyRelTol=0.001  ConsistencyTolFactor=0.001  UseLocalSolver=off  LocalSolverChoice=NE_BACKWARD_EULER_ADVANCER  ResolveIndetEquations=on  FunctionEvalNumThread=1  LocalSolverSampleTime=0.001  DoFixedCost=off  MaxNonlinIter=3  MaxModeIter=2  ComputeImpulses=off  ImpulseIterations=2  LinearAlgebra=Sparse  LinearAlgebraNumThread=0  EquationFormulation=NE_TIME_EF  DelaysMemoryBudget=1024  AutomaticFiltering=on  FilteringTimeConstant=0.001  PartitionStorageMethod=AS_NEEDED  PartitionMemoryBudget=1024  PartitionMethod=FAST  MultibodyUseLocalSolver=off  MultibodyLocalSolverChoice=ODE1  MultibodyLocalSolverSampleTime=0.001
  C : PMIOPort  Side=Right
  connections:
  Mechanism Configuration/RConn1 -- Solver Configuration/RConn1 -- C/RConn1

== matlab function SBCAFinalSim/MATLAB Function1 ==
  settings: updateMethod=DISCRETE
  data: R_corner input; R_desired output; omega input; data input; R_current input
function R_desired = despool_tilt_controller(R_corner, omega, data, R_current)
% despool_tilt_controller - Tilt R_corner up to 10 deg in direction of omega*R_current
%
% Inputs:
%   R_corner  - 3x3 rotation matrix of cube balanced on corner (fixed setpoint)
%   omega     - 3x1 angular velocity vector in body frame
%   R_current - 3x3 current rotation matrix (body-to-world)
%
% Output:
%   R_desired - 3x3 desired rotation matrix (tilted setpoint)

    % Apply bias to omega
    omega = omega -[-0.1;0.1;-0.1];
    persistent omega_smooth initialized
alpha = 0.005;  % smoothing factor (tune between 0.005)

if isempty(initialized)
    omega_smooth = omega;   % initialize
    initialized = true;
end

omega_smooth = (1 - alpha) * omega_smooth + alpha * omega;

omega = omega_smooth; 
%omega=omega-mean(omega);
omega = sign(omega).*abs(omega).^2+omega;
omega = max(min(omega, 0.4), -0.4);
    

    tilt_axis_world =  eulerToR(omega/2);

    R_desired = tilt_axis_world  * R_corner;
end

function R = axisAngleToRotationMatrix(axis, angle)
    % Rodrigues' rotation formula
    axis = axis / norm(axis);
    K = [  0       -axis(3)  axis(2);
          axis(3)     0     -axis(1);
         -axis(2)  axis(1)     0  ];
    R = eye(3) + sin(angle) * K + (1 - cos(angle)) * (K * K);
end
function R = eulerToR(omega)
% omega = [roll; pitch; yaw] in radians

    roll  = omega(1);
    pitch = omega(2);
    yaw   = omega(3);

    Rx = [1, 0, 0;
          0, cos(roll), -sin(roll);
          0, sin(roll),  cos(roll)];

    Ry = [ cos(pitch), 0, sin(pitch);
           0, 1, 0;
          -sin(pitch), 0, cos(pitch)];

    Rz = [cos(yaw), -sin(yaw), 0;
          sin(yaw),  cos(yaw), 0;
          0, 0, 1];

    % Final combined rotation
    R = Rz * Ry * Rx;
end

== matlab function SBCAFinalSim/MATLAB Function ==
  settings: updateMethod=DISCRETE
  data: R input; R_desired input; omega input; tau output; K1 input; K2 input; data input
function tau = balanceCubeLQR(R, R_desired, omega, K1, K2, data)
% balanceCubeLQR - Computes torque using angle-dependent LQR with smooth transition
%
% Inputs:
%   R         - Current rotation matrix (3x3)
%   R_desired - Desired rotation matrix (3x3)
%   omega     - Angular velocity in body frame (3x1)
%   K1        - LQR gain matrix for small error (3x6)
%   K2        - LQR gain matrix for large error (3x6)
%
% Output:
%   tau       - Torque command (3x1)

    % Compute state vector
    x = computeStateVector(R, R_desired, omega);

    % --- Compute misalignment angle between R and R_desired ---
    R_err = R_desired' * R;
    cos_theta = (trace(R_err) - 1) / 2;
    cos_theta = max(min(cos_theta, 1), -1);  % numerical safety
    angle_err_mag = acosd(cos_theta);        % in degrees

    % --- Blended gain selection ---
    if angle_err_mag <= 10
        alpha = 0;   % fully K1
    elseif angle_err_mag >= 25
        alpha = 1;   % fully K2
    else
        % Linear blend between 5° and 10°
        alpha = (angle_err_mag - 10) / 15;
    end


    

    % --- LQR torque command ---
    tau = -K1 * x.*alpha-K2*x.*(1-alpha);%+[0.05;-0.05;0.05];

    % --- Torque saturation ---
    max_tau = 1;  % Adjust based on motor/wheel limits
    tau = max(min(tau, max_tau), -max_tau);
    alpha1 = 0.5;
    persistent tau_prev
if isempty(tau_prev)
    tau_prev = zeros(size(tau));
end

tau_out = tau;
for i = 1:numel(tau)
    if abs(tau) < abs(tau_prev)
        tau_out = alpha1 * tau + (1 - alpha1) * tau_prev;
    end
end
tau=tau_out;
%tau(3)=0;
%tau(1)=0;
tau_prev = tau_out;
end

%% Helper functions
function x = computeStateVector(R, R_desired, omega)
    % Computes the 6x1 state vector [angle_error; angular_velocity]
    R_err = R_desired' * R;
    angle_err = vee(R_err - R_err') / 2;
    x = [angle_err; omega];
end

function v = vee(S)
    % Maps a skew-symmetric matrix to a 3x1 vector
    v = [S(3,2); S(1,3); S(2,1)];
end

== matlab function SBCAFinalSim/MATLAB Function2 ==
  data: R_corner output; x input
function R_corner= computeTiltedRDesired(x)
    % Rotation of 90 degrees about the y-axis
    theta = pi/4;  % 90 degrees in radians
    R_edge = [ cos(theta),  0, sin(theta);
               0,           1, 0;
              -sin(theta),  0, cos(theta) ];




       % --- Corner orientation ---
    corner_body = [1; 1; 1];
    z_hat = corner_body / norm(corner_body);
    
    helper = [1; 0; 0];
    if abs(dot(helper, z_hat)) > 0.9
        helper = [0; 1; 0];
    end

    y_hat = cross(z_hat, helper);
    y_hat = y_hat / norm(y_hat);
    x_hat = cross(y_hat, z_hat);

    R_corner = [x_hat, y_hat, z_hat];  % corner-to-world rotation
   
       % R_corner=R_edge;
  


end

== matlab function SBCAFinalSim/MATLAB Function3 ==
  data: duty input; tau_motor output; omega_w input
function tau_motor = ESC_Motor(duty, omega_w)
% ESC_Motor - More realistic BLDC motor + ESC model
% Inputs:
%   duty    - ESC command [0..1] (normalized throttle)
%   omega_w - motor angular velocity [rad/s]
% Output:
%   tau_motor - motor torque [Nm]

% ================= Motor/ESC parameters =================
Vbatt  = 11.5;           % 3S LiPo nominal voltage (V)
kV     = 920;             % RPM per Volt
R      = 0.3;             % Phase resistance (Ohm)
Kt     = 60/(2*pi*kV);    % Torque constant (Nm/A)
Ke     = Kt;              % Back EMF constant (V·s/rad)
I_max  = 30;              % Max ESC/motor current (A)
tau_max = Kt * I_max;     % Max torque (Nm)

% Non-ideal ESC mapping (deadband + nonlinearity)
% Apply deadband around zero
if abs(duty) < 0.05
    duty_eff = 0;  
else
    % Rescale so that after deadband, it maps back to [-1,1]
    duty_eff = (abs(duty) - 0.05) / (1 - 0.05);  
    duty_eff = sign(duty) * duty_eff;  % restore original sign
end

% Clamp to [-1,1]
duty_eff = min(max(duty, -1), 1);

% Effective applied motor voltage
V_m = duty_eff * Vbatt;

% ================= Motor electrical model =================
I = (V_m - Ke*omega_w) / R;   % phase current

% Saturate current (ESC current limit)
I = max(min(I, I_max), -I_max);

% Electromagnetic torque
tau_e = Kt * I;

% ================= Losses =================
tau_visc = 1e-4 * omega_w;     % viscous friction (linear)
tau_drag = 1e-6 * omega_w^2;   % aerodynamic/rotor drag (quadratic)

% ================= Net torque =================
tau_motor = tau_e ;

% Saturate torque
tau_motor = max(min(tau_motor, tau_max), -tau_max);

end

== matlab function SBCAFinalSim/MATLAB Function4 ==
  data: duty input; tau_motor output; omega_w input
function tau_motor = ESC_Motor(duty, omega_w)
% ESC_Motor - More realistic BLDC motor + ESC model
% Inputs:
%   duty    - ESC command [0..1] (normalized throttle)
%   omega_w - motor angular velocity [rad/s]
% Output:
%   tau_motor - motor torque [Nm]

% ================= Motor/ESC parameters =================
Vbatt  = 11.5;           % 3S LiPo nominal voltage (V)
kV     = 920;             % RPM per Volt
R      = 0.3;             % Phase resistance (Ohm)
Kt     = 60/(2*pi*kV);    % Torque constant (Nm/A)
Ke     = Kt;              % Back EMF constant (V·s/rad)
I_max  = 30;              % Max ESC/motor current (A)
tau_max = Kt * I_max;     % Max torque (Nm)

% Non-ideal ESC mapping (deadband + nonlinearity)
% Apply deadband around zero
if abs(duty) < 0.05
    duty_eff = 0;  
else
    % Rescale so that after deadband, it maps back to [-1,1]
    duty_eff = (abs(duty) - 0.05) / (1 - 0.05);  
    duty_eff = sign(duty) * duty_eff;  % restore original sign
end

% Clamp to [-1,1]
duty_eff = min(max(duty, -1), 1);

% Effective applied motor voltage
V_m = duty_eff * Vbatt;

% ================= Motor electrical model =================
I = (V_m - Ke*omega_w) / R;   % phase current

% Saturate current (ESC current limit)
I = max(min(I, I_max), -I_max);

% Electromagnetic torque
tau_e = Kt * I;

% ================= Losses =================
tau_visc = 1e-4 * omega_w;     % viscous friction (linear)
tau_drag = 1e-6 * omega_w^2;   % aerodynamic/rotor drag (quadratic)

% ================= Net torque =================
tau_motor = tau_e ;

% Saturate torque
tau_motor = max(min(tau_motor, tau_max), -tau_max);

end

== matlab function SBCAFinalSim/MATLAB Function5 ==
  data: duty input; tau_motor output; omega_w input
function tau_motor = ESC_Motor(duty, omega_w)
% ESC_Motor - More realistic BLDC motor + ESC model
% Inputs:
%   duty    - ESC command [0..1] (normalized throttle)
%   omega_w - motor angular velocity [rad/s]
% Output:
%   tau_motor - motor torque [Nm]

% ================= Motor/ESC parameters =================
Vbatt  = 11.5;           % 3S LiPo nominal voltage (V)
kV     = 920;             % RPM per Volt
R      = 0.3;             % Phase resistance (Ohm)
Kt     = 60/(2*pi*kV);    % Torque constant (Nm/A)
Ke     = Kt;              % Back EMF constant (V·s/rad)
I_max  = 30;              % Max ESC/motor current (A)
tau_max = Kt * I_max;     % Max torque (Nm)

% Non-ideal ESC mapping (deadband + nonlinearity)
% Apply deadband around zero
if abs(duty) < 0.05
    duty_eff = 0;  
else
    % Rescale so that after deadband, it maps back to [-1,1]
    duty_eff = (abs(duty) - 0.05) / (1 - 0.05);  
    duty_eff = sign(duty) * duty_eff;  % restore original sign
end

% Clamp to [-1,1]
duty_eff = min(max(duty, -1), 1);

% Effective applied motor voltage
V_m = duty_eff * Vbatt;

% ================= Motor electrical model =================
I = (V_m - Ke*omega_w) / R;   % phase current

% Saturate current (ESC current limit)
I = max(min(I, I_max), -I_max);

% Electromagnetic torque
tau_e = Kt * I;

% ================= Losses =================
tau_visc = 1e-4 * omega_w;     % viscous friction (linear)
tau_drag = 1e-6 * omega_w^2;   % aerodynamic/rotor drag (quadratic)

% ================= Net torque =================
tau_motor = tau_e ;

% Saturate torque
tau_motor = max(min(tau_motor, tau_max), -tau_max);

end

== matlab function SBCAFinalSim/MATLAB Function6 ==
  data: R input; q output
function q = rotm2quat(R)
% ROTM2QUAT Converts a 3x3 rotation matrix to a quaternion.
%
%   q = ROTM2QUAT(R)
%
% Inputs:
%   R - 3x3 rotation matrix (must be orthonormal and det(R) ≈ 1)
%
% Outputs:
%   q - 1x4 quaternion [w, x, y, z], where:
%       w is the scalar part
%       x, y, z are the vector parts
%
% Notes:
%   - The function ensures numerical stability by choosing the largest
%     diagonal element of R to determine which component of q to compute first.
%   - Assumes right-handed coordinate system.

    % Ensure R is valid
    if ~isequal(size(R), [3, 3])
        error('Input must be a 3x3 rotation matrix.');
    end

    tr = trace(R);

    if tr > 0
        S = sqrt(tr + 1.0) * 2; % S = 4 * qw
        qw = 0.25 * S;
        qx = (R(3,2) - R(2,3)) / S;
        qy = (R(1,3) - R(3,1)) / S;
        qz = (R(2,1) - R(1,2)) / S;
    elseif (R(1,1) > R(2,2)) && (R(1,1) > R(3,3))
        S = sqrt(1.0 + R(1,1) - R(2,2) - R(3,3)) * 2; % S = 4 * qx
        qw = (R(3,2) - R(2,3)) / S;
        qx = 0.25 * S;
        qy = (R(1,2) + R(2,1)) / S;
        qz = (R(1,3) + R(3,1)) / S;
    elseif R(2,2) > R(3,3)
        S = sqrt(1.0 + R(2,2) - R(1,1) - R(3,3)) * 2; % S = 4 * qy
        qw = (R(1,3) - R(3,1)) / S;
        qx = (R(1,2) + R(2,1)) / S;
        qy = 0.25 * S;
        qz = (R(2,3) + R(3,2)) / S;
    else
        S = sqrt(1.0 + R(3,3) - R(1,1) - R(2,2)) * 2; % S = 4 * qz
        qw = (R(2,1) - R(1,2)) / S;
        qx = (R(1,3) + R(3,1)) / S;
        qy = (R(2,3) + R(3,2)) / S;
        qz = 0.25 * S;
    end

    % Normalize to ensure unit quaternion
    q = [qw, qx, qy, qz];
    q = q / norm(q);

end

== matlab function SBCAFinalSim/MATLAB Function7 ==
  data: R input; q output
function q = rotm2quat(R)
% ROTM2QUAT Converts a 3x3 rotation matrix to a quaternion.
%
%   q = ROTM2QUAT(R)
%
% Inputs:
%   R - 3x3 rotation matrix (must be orthonormal and det(R) ≈ 1)
%
% Outputs:
%   q - 1x4 quaternion [w, x, y, z], where:
%       w is the scalar part
%       x, y, z are the vector parts
%
% Notes:
%   - The function ensures numerical stability by choosing the largest
%     diagonal element of R to determine which component of q to compute first.
%   - Assumes right-handed coordinate system.

    % Ensure R is valid
    if ~isequal(size(R), [3, 3])
        error('Input must be a 3x3 rotation matrix.');
    end

    tr = trace(R);

    if tr > 0
        S = sqrt(tr + 1.0) * 2; % S = 4 * qw
        qw = 0.25 * S;
        qx = (R(3,2) - R(2,3)) / S;
        qy = (R(1,3) - R(3,1)) / S;
        qz = (R(2,1) - R(1,2)) / S;
    elseif (R(1,1) > R(2,2)) && (R(1,1) > R(3,3))
        S = sqrt(1.0 + R(1,1) - R(2,2) - R(3,3)) * 2; % S = 4 * qx
        qw = (R(3,2) - R(2,3)) / S;
        qx = 0.25 * S;
        qy = (R(1,2) + R(2,1)) / S;
        qz = (R(1,3) + R(3,1)) / S;
    elseif R(2,2) > R(3,3)
        S = sqrt(1.0 + R(2,2) - R(1,1) - R(3,3)) * 2; % S = 4 * qy
        qw = (R(1,3) - R(3,1)) / S;
        qx = (R(1,2) + R(2,1)) / S;
        qy = 0.25 * S;
        qz = (R(2,3) + R(3,2)) / S;
    else
        S = sqrt(1.0 + R(3,3) - R(1,1) - R(2,2)) * 2; % S = 4 * qz
        qw = (R(2,1) - R(1,2)) / S;
        qx = (R(1,3) + R(3,1)) / S;
        qy = (R(2,3) + R(3,2)) / S;
        qz = 0.25 * S;
    end

    % Normalize to ensure unit quaternion
    q = [qw, qx, qy, qz];
    q = q / norm(q);

end
